simulink model "FreqDomainControl"  (R2015a)
settings: Solver=ode45  StartTime=0.0  StopTime=10.0  RelTol=1e-3
settings Model: NumberOfSteps=2  Creator=khalil  LastModifiedBy=khalil

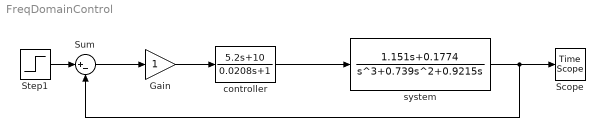
== system FreqDomainControl ==
  Gain : Gain
  Scope : TimeScope
  Step1 : Step  Time=.01  SampleTime=0
  Sum : Sum  Inputs=|+-
  controller : TransferFcn  Numerator=[5.2,10]  Denominator=[0.0208,1]
  system : TransferFcn  Numerator=[1.151,0.1774]  Denominator=[1,0.739,0.9215,0]
  wires:
  controller/1 -> system/1
  system/1 -> Sum/2, Scope/1
  Sum/1 -> Gain/1
  Step1/1 -> Sum/1
  Gain/1 -> controller/1
